simulink model "duo_waveadder"  (R2021a)
settings: Solver=FixedStepAuto  StartTime=0.0  StopTime=10.0  FixedStep=0.001  RelTol=1e-3
settings Model: Creator=Davie  LastModifiedBy=Davie

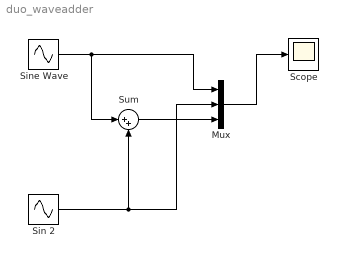
== system duo_waveadder ==
  Mux : Mux  Inputs=3
  Scope : Scope
  Sin 2 : Sin  Frequency=258  SampleTime=0
  Sine Wave : Sin  Frequency=256  SampleTime=0
  Sum : Sum  Inputs=|++
  wires:
  Sine Wave/1 -> Sum/1, Mux/1
  Sin 2/1 -> Mux/2, Sum/2
  Sum/1 -> Mux/3
  Mux/1 -> Scope/1
